simulink model "Subsystem"  (R2017a)
settings: Solver=VariableStepAuto  StartTime=0.0  StopTime=tf  FixedStep=1e-4  RelTol=1e-5
values from neighbouring files (symbols this model uses):
  x0 = [0; 0]    [load_motor_params.m]
undefined symbols (not defined in the file or in its folder): A, B, C_, Ctilde, mean_val, Tpwm_val, Ts_val, var_val, Vcc_val
settings Model: Creator=brunolnetto  LastModifiedBy=brunolnetto
settings DataIOCC: SaveOutput=off  SaveTime=off

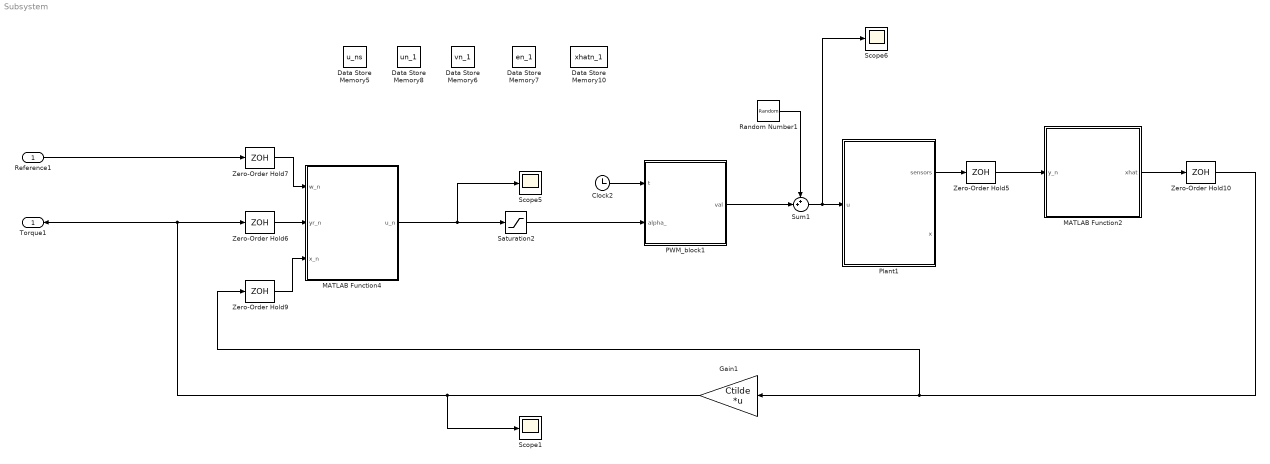
== system Subsystem ==
  Reference1 : Inport  OutDataTypeStr=double  PortDimensions=1  SampleTime=[0.01,0]
  Clock2 : Clock
  Data Store Memory10 : DataStoreMemory  DataStoreName=xhatn_1  InitialValue=xhat0  ShowAdditionalParam=off  OutDataTypeStr=double
  Data Store Memory5 : DataStoreMemory  DataStoreName=u_ns  InitialValue=u_ns0  ShowAdditionalParam=off  OutDataTypeStr=double
  Data Store Memory6 : DataStoreMemory  DataStoreName=vn_1  ShowAdditionalParam=off  OutDataTypeStr=double
  Data Store Memory7 : DataStoreMemory  DataStoreName=en_1  InitialValue=e0  ShowAdditionalParam=off  OutDataTypeStr=double
  Data Store Memory8 : DataStoreMemory  DataStoreName=un_1  ReadBeforeWriteMsg=warning  WriteAfterWriteMsg=warning  WriteAfterReadMsg=warning  ShowAdditionalParam=off  OutDataTypeStr=double
  Gain1 : Gain  Gain=Ctilde  Multiplication=Matrix(K*u) (u vector)
  MATLAB Function2 : MATLAB Function  TreatAsAtomicUnit=on
  MATLAB Function4 : MATLAB Function  TreatAsAtomicUnit=on
  PWM_block1 : MATLAB Function  TreatAsAtomicUnit=on
  Plant1 : Subsystem
  Random Number1 : RandomNumber  Mean=mean_val  Variance=var_val  SampleTime=Ts_val
  Saturation2 : Saturate  UpperLimit=1  LowerLimit=-1
  Scope1 : Scope
  Scope5 : Scope
  Scope6 : Scope
  Sum1 : Sum  Inputs=++|
  Zero-Order Hold{5..7,9..10} (5 alike) : ZeroOrderHold  SampleTime=Ts_val
  Torque1 : Outport  OutDataTypeStr=double  PortDimensions=1  SampleTime=[0.01,0]
  wires:
  Plant1/1(sensors) -> Zero-Order Hold5/1
  Zero-Order Hold6/1 -> MATLAB Function4/2(yr_n)
  PWM_block1/1(val) -> Sum1/2
  Random Number1/1 -> Sum1/1
  Sum1/1 -> Scope6/1, Plant1/1(u)
  Reference1/1 -> Zero-Order Hold7/1
  Zero-Order Hold5/1 -> MATLAB Function2/1(y_n)
  Clock2/1 -> PWM_block1/1(t)
  MATLAB Function2/1(xhat) -> Zero-Order Hold10/1
  Saturation2/1 -> PWM_block1/2(alpha_)
  MATLAB Function4/1(u_n) -> Scope5/1, Saturation2/1
  Zero-Order Hold10/1 -> Zero-Order Hold9/1, Gain1/1
  Zero-Order Hold9/1 -> MATLAB Function4/3(x_n)
  Zero-Order Hold7/1 -> MATLAB Function4/1(w_n)
  Gain1/1 -> Scope1/1, Torque1/1, Zero-Order Hold6/1

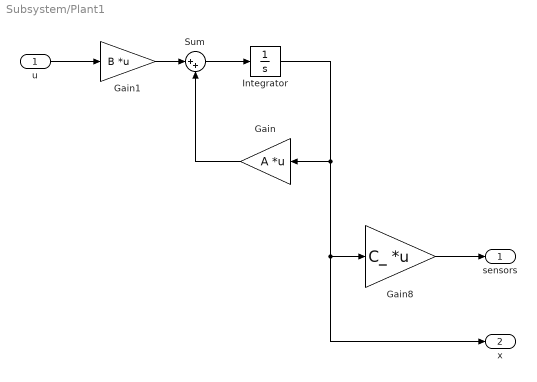
== system Subsystem/Plant1 ==
  u : Inport
  Gain : Gain  Gain=A  Multiplication=Matrix(K*u) (u vector)
  Gain1 : Gain  Gain=B  Multiplication=Matrix(K*u) (u vector)
  Gain8 : Gain  Gain=C_  Multiplication=Matrix(K*u) (u vector)
  Integrator : Integrator  InitialCondition=x0
  Sum : Sum  Inputs=|++
  sensors : Outport
  x : Outport  Port=2
  wires:
  Gain8/1 -> sensors/1
  Gain1/1 -> Sum/1
  u/1 -> Gain1/1
  Gain/1 -> Sum/2
  Sum/1 -> Integrator/1
  Integrator/1 -> x/1, Gain8/1, Gain/1

== matlab function Subsystem/MATLAB Function2 ==
  data: y_n input; xhat output; un_1 data_store_memory; xhatn_1 data_store_memory; params parameter
function xhat = observador (y_n, params)
    global un_1;
    global xhatn_1;
    
%     x_bar = params.Phi*xhatn_1 + params.Gamma*un_1;
%     xhat = x_bar + params.L*(y - params.C*xhatn_1);
    
    Phi = params.Phi;
    Gamma = params.Gamma;
    L = params.L;
    C = params.C;

    xhat = Phi*xhatn_1 + Gamma*un_1 + L*(y_n - C*xhatn_1);

    xhatn_1 = xhat;
end

== matlab function Subsystem/MATLAB Function4 ==
  data: w_n input; yr_n input; x_n input; u_n output; vn_1 data_store_memory; params parameter; en_1 data_store_memory; un_1 data_store_memory; u_ns data_store_memory
function u_n = controller(w_n, yr_n, x_n, params)
    global vn_1;
    global en_1;
    global un_1;
    global u_ns;
    
    x_n = [x_n; u_ns];    
    v_n = vn_1 + en_1;
    
    u_i = params.Ki*v_n;
    u_p = - params.Kp*x_n;
    
    u_n = u_i + u_p;
    
    vn_1 = v_n;
    en_1 = w_n - yr_n;
    un_1 = u_n;
    u_ns = [u_n; u_ns(2:end)];
end

== matlab function Subsystem/PWM_block1 ==
  data: t input; alpha_ input; val output; Vcc_val parameter; Tpwm_val parameter
function val = pwm_signal(t, alpha_, Vcc_val, Tpwm_val)
    % Static variable
    persistent t0;
    
    if(isempty(t0))
        t0 = 0;
    end
        
    % PWM generation
    if(t == 0)
        t0 = 0;
    end
    
    if(t - t0 > Tpwm_val)
        t0 = t;
    end
    
    % Inner time interval
    t_i = t - t0;
    
    abs_alpha = abs(alpha_);
    sign_alpha = sign(alpha_);
    
    if(t_i <= abs_alpha*Tpwm_val)
        val = sign_alpha*Vcc_val;
    else
        val = 0;
    end
end
